simulink model "ResolverOffsetCalibrationComponent"  (R2025b)
settings: Solver=FixedStepDiscrete  StartTime=0.0  StopTime=10.0  RelTol=1e-3
settings Model: DataDictionary=TractionEmotorSoftwareArchInterfaceData.sldd  Creator=dakaihu  LastModifiedBy=dakaihu
settings OptimizationCC: ReuseModelBlockBuffer=off
settings RTWCC: GPUComputeCapability=3.5

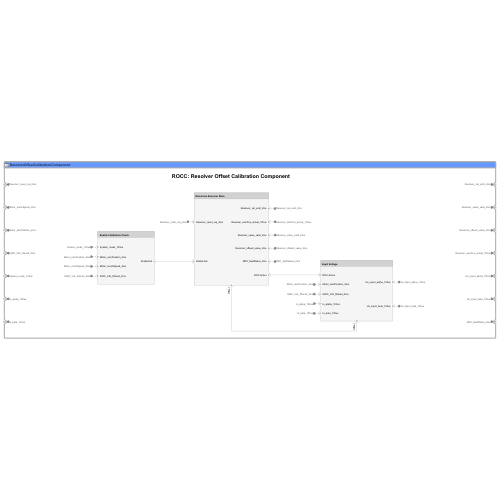
[thumbnail: Simulink's stored preview of the top-level diagram]
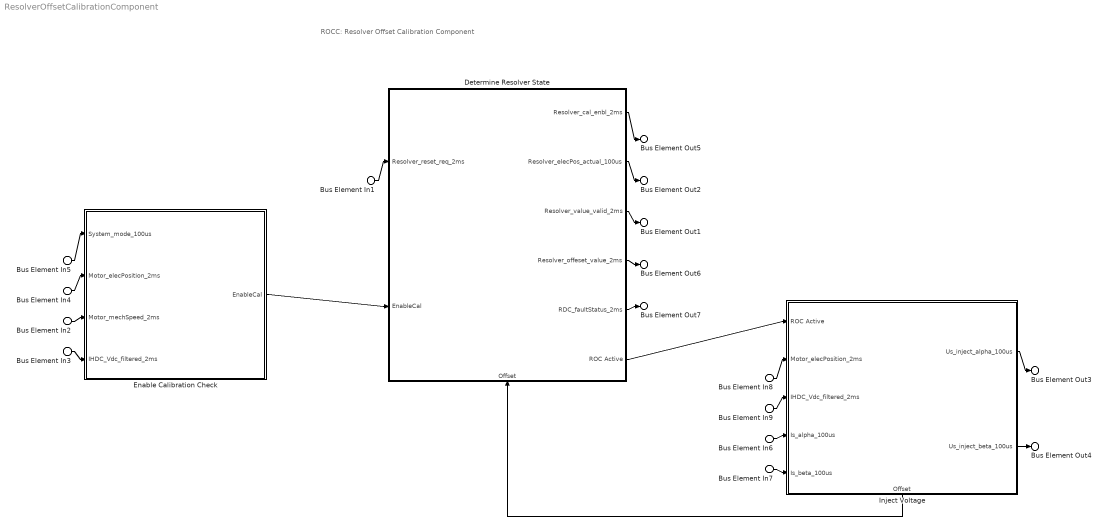
== system ResolverOffsetCalibrationComponent ==
  note: ROCC: Resolver Offset Calibration Component
  Bus Element In1 : Inport  PortName=Resolver_reset_req_2ms
  Bus Element In2 : Inport  Port=2  PortName=Motor_mechSpeed_2ms
  Bus Element In4 : Inport  Port=3  PortName=Motor_elecPosition_2ms
  Bus Element In8 : Inport  Port=3  PortName=Motor_elecPosition_2ms
  Bus Element In3 : Inport  Port=4  PortName=IHDC_Vdc_filtered_2ms
  Bus Element In9 : Inport  Port=4  PortName=IHDC_Vdc_filtered_2ms
  Bus Element In5 : Inport  Port=5  PortName=System_mode_100us
  Bus Element In6 : Inport  Port=6  PortName=Is_alpha_100us
  Bus Element In7 : Inport  Port=7  PortName=Is_beta_100us
  " Enable Calibration Check" : Subsystem
      settings: PortSchema="{\"entries\":[{\"content\":{\"headerSize\":26,\"margin\":15,\"minimumSpacing\":25,\"sides\":[{\"content\":{\"connectorIds\":[\"In1\",\"In2\",\"In3\",\"In4\"]},\"type\":\"ConnectorPlacement.EquallySpacedRectSide\",\"uuid\":\"a0c63ab2-75fe-4bec-b2b0-6e2e00a1a5a4\"},{\"content\":{\"connectorIds\":[\"Out1\"],\"side\":\"RIGHT\"},\"type\":\"ConnectorPlacement.EquallySpacedRectSide\",\"uuid\":\"05d605ea-8968-4533-a01c-bf4aae5caa93\"},{\"content\":{\"connectorIds\":[],\"side\":\"TOP\"},\"type\":\"ConnectorPlacement.EquallySpacedRectSide\",\"uuid\":\"27167c69-3967-4107-acce-f317c3d854af\"}]},\"type\":\"ConnectorPlacement.EquallySpacedConnector\",\"uuid\":\"c4d90da2-0f2a-4c00-bd24-85fead00d18f\"}],\"packageUris\":[\"http://schema.mathworks.com/mf0/Connector/R2020b\"],\"version\":\"1.0\"}"
  Determine Resolver State : Subsystem
      settings: PortSchema="{\"entries\":[{\"content\":{\"headerSize\":26,\"margin\":15,\"minimumSpacing\":25,\"sides\":[{\"content\":{\"connectorIds\":[\"In1\",\"In3\"]},\"type\":\"ConnectorPlacement.EquallySpacedRectSide\",\"uuid\":\"a0c63ab2-75fe-4bec-b2b0-6e2e00a1a5a4\"},{\"content\":{\"connectorIds\":[\"Out1\",\"Out2\",\"Out3\",\"Out4\",\"Out5\",\"Out6\"],\"side\":\"RIGHT\"},\"type\":\"ConnectorPlacement.EquallySpacedRectSide\",\"uuid\":\"05d605ea-8968-4533-a01c-bf4aae5caa93\"},{\"content\":{\"connectorIds\":[],\"side\":\"TOP\"},\"type\":\"ConnectorPlacement.EquallySpacedRectSide\",\"uuid\":\"27167c69-3967-4107-acce-f317c3d854af\"},{\"content\":{\"connectorIds\":[\"In2\"],\"side\":\"BOTTOM\"},\"type\":\"ConnectorPlacement.EquallySpacedRectSide\",\"uuid\":\"c9b74918-598e-400e-b426-c23497545141\"}]},\"type\":\"ConnectorPlacement.EquallySpacedConnector\",\"uuid\":\"c4d90da2-0f2a-4c00-bd24-85fead00d18f\"}],\"packageUris\":[\"http://schema.mathworks.com/mf0/Connector/R2020b\"],\"version\":\"1.0\"}"
  Inject Voltage : Subsystem
      settings: PortSchema="{\"entries\":[{\"content\":{\"headerSize\":26,\"margin\":15,\"minimumSpacing\":25,\"sides\":[{\"content\":{\"connectorIds\":[\"In1\",\"In2\",\"In3\",\"In4\",\"In5\"]},\"type\":\"ConnectorPlacement.EquallySpacedRectSide\",\"uuid\":\"a0c63ab2-75fe-4bec-b2b0-6e2e00a1a5a4\"},{\"content\":{\"connectorIds\":[\"Out1\",\"Out2\"],\"side\":\"RIGHT\"},\"type\":\"ConnectorPlacement.EquallySpacedRectSide\",\"uuid\":\"05d605ea-8968-4533-a01c-bf4aae5caa93\"},{\"content\":{\"connectorIds\":[],\"side\":\"TOP\"},\"type\":\"ConnectorPlacement.EquallySpacedRectSide\",\"uuid\":\"27167c69-3967-4107-acce-f317c3d854af\"},{\"content\":{\"connectorIds\":[\"Out3\"],\"side\":\"BOTTOM\"},\"type\":\"ConnectorPlacement.EquallySpacedRectSide\",\"uuid\":\"5a7584c0-1216-42bf-b1d4-90b9a06c8ab4\"}]},\"type\":\"ConnectorPlacement.EquallySpacedConnector\",\"uuid\":\"c4d90da2-0f2a-4c00-bd24-85fead00d18f\"}],\"packageUris\":[\"http://schema.mathworks.com/mf0/Connector/R2020b\"],\"version\":\"1.0\"}"
  Bus Element Out5 : Outport  PortName=Resolver_cal_enbl_2ms
  Bus Element Out1 : Outport  Port=2  PortName=Resolver_value_valid_2ms
  Bus Element Out6 : Outport  Port=3  PortName=Resolver_offeset_value_2ms
  Bus Element Out2 : Outport  Port=4  PortName=Resolver_elecPos_actual_100us
  Bus Element Out3 : Outport  Port=5  PortName=Us_inject_alpha_100us
  Bus Element Out4 : Outport  Port=6  PortName=Us_inject_beta_100us
  Bus Element Out7 : Outport  Port=7  PortName=RDC_faultStatus_2ms
  wires:
  " Enable Calibration Check"/1(EnableCal) -> Determine Resolver State/3(EnableCal)
  Bus Element In2/1 -> " Enable Calibration Check"/3(Motor_mechSpeed_2ms)
  Bus Element In4/1 -> " Enable Calibration Check"/2(Motor_elecPosition_2ms)
  Bus Element In3/1 -> " Enable Calibration Check"/4(IHDC_Vdc_filtered_2ms)
  Bus Element In5/1 -> " Enable Calibration Check"/1(System_mode_100us)
  Determine Resolver State/6(ROC Active) -> Inject Voltage/1(ROC Active)
  Bus Element In8/1 -> Inject Voltage/2(Motor_elecPosition_2ms)
  Bus Element In9/1 -> Inject Voltage/3(IHDC_Vdc_filtered_2ms)
  Bus Element In6/1 -> Inject Voltage/4(Is_alpha_100us)
  Bus Element In7/1 -> Inject Voltage/5(Is_beta_100us)
  Inject Voltage/3(Offset) -> Determine Resolver State/2(Offset)
  Inject Voltage/1(Us_inject_alpha_100us) -> Bus Element Out3/1
  Inject Voltage/2(Us_inject_beta_100us) -> Bus Element Out4/1
  Determine Resolver State/1(Resolver_cal_enbl_2ms) -> Bus Element Out5/1
  Determine Resolver State/2(Resolver_elecPos_actual_100us) -> Bus Element Out2/1
  Determine Resolver State/3(Resolver_value_valid_2ms) -> Bus Element Out1/1
  Determine Resolver State/4(Resolver_offeset_value_2ms) -> Bus Element Out6/1
  Determine Resolver State/5(RDC_faultStatus_2ms) -> Bus Element Out7/1
  Bus Element In1/1 -> Determine Resolver State/1(Resolver_reset_req_2ms)

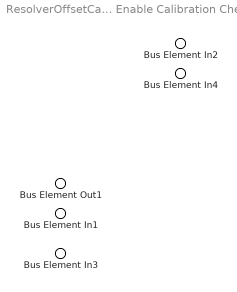
== system ResolverOffsetCalibrationComponent/ Enable Calibration Check ==
  Bus Element In4 : Inport  PortName=System_mode_100us
  Bus Element In2 : Inport  Port=2  PortName=Motor_elecPosition_2ms
  Bus Element In1 : Inport  Port=3  PortName=Motor_mechSpeed_2ms
  Bus Element In3 : Inport  Port=4  PortName=IHDC_Vdc_filtered_2ms
  Bus Element Out1 : Outport  PortName=EnableCal

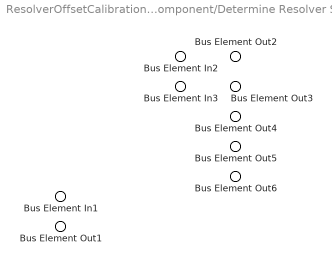
== system ResolverOffsetCalibrationComponent/Determine Resolver State ==
  Bus Element In3 : Inport  PortName=Resolver_reset_req_2ms
  Bus Element In2 : Inport  Port=2  PortName=Offset
  Bus Element In1 : Inport  Port=3  PortName=EnableCal
  Bus Element Out2 : Outport  PortName=Resolver_cal_enbl_2ms
  Bus Element Out3 : Outport  Port=2  PortName=Resolver_elecPos_actual_100us
  Bus Element Out4 : Outport  Port=3  PortName=Resolver_value_valid_2ms
  Bus Element Out5 : Outport  Port=4  PortName=Resolver_offeset_value_2ms
  Bus Element Out6 : Outport  Port=5  PortName=RDC_faultStatus_2ms
  Bus Element Out1 : Outport  Port=6  PortName=ROC Active

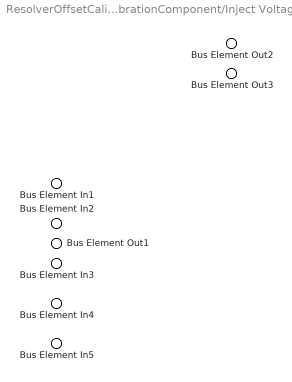
== system ResolverOffsetCalibrationComponent/Inject Voltage ==
  Bus Element In1 : Inport  PortName=ROC Active
  Bus Element In2 : Inport  Port=2  PortName=Motor_elecPosition_2ms
  Bus Element In3 : Inport  Port=3  PortName=IHDC_Vdc_filtered_2ms
  Bus Element In4 : Inport  Port=4  PortName=Is_alpha_100us
  Bus Element In5 : Inport  Port=5  PortName=Is_beta_100us
  Bus Element Out2 : Outport  PortName=Us_inject_alpha_100us
  Bus Element Out3 : Outport  Port=2  PortName=Us_inject_beta_100us
  Bus Element Out1 : Outport  Port=3  PortName=Offset
